simulink model "SysErrorDetect"  (R2019a)
settings: Solver=VariableStepAuto  StartTime=0.0  StopTime=10.0  RelTol=1e-3
settings Model: Creator=arsp2701  LastModifiedBy=arsp2701

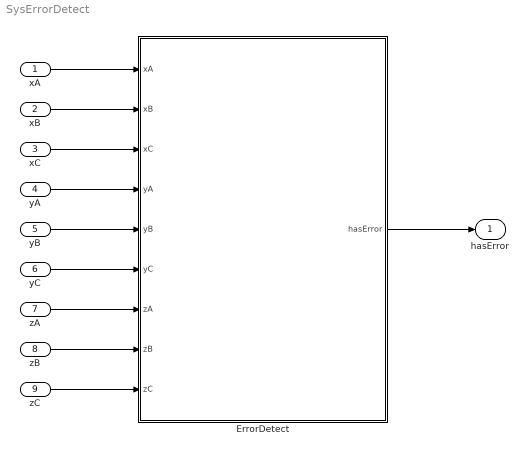
== system SysErrorDetect ==
  xA : Inport
  xB : Inport  Port=2
  xC : Inport  Port=3
  yA : Inport  Port=4
  yB : Inport  Port=5
  yC : Inport  Port=6
  zA : Inport  Port=7
  zB : Inport  Port=8
  zC : Inport  Port=9
  ErrorDetect : MATLAB Function  TreatAsAtomicUnit=on
  hasError : Outport
  wires:
  ErrorDetect/1(hasError) -> hasError/1
  xA/1 -> ErrorDetect/1(xA)
  xB/1 -> ErrorDetect/2(xB)
  xC/1 -> ErrorDetect/3(xC)
  yA/1 -> ErrorDetect/4(yA)
  yB/1 -> ErrorDetect/5(yB)
  yC/1 -> ErrorDetect/6(yC)
  zA/1 -> ErrorDetect/7(zA)
  zB/1 -> ErrorDetect/8(zB)
  zC/1 -> ErrorDetect/9(zC)

== matlab function SysErrorDetect/ErrorDetect ==
  data: xA input; xB input; hasError output; xC input; yA input; yB input; yC input; zA input; zB input; zC input
function hasError = ErrorDetect(xA, xB, xC, yA, yB, yC, zA, zB, zC)
    % Compute phi and theta (page 23)
    T_ABC = [
        yA -xA 1;
        yB -xB 1;
        yC -xC 1;
    ];
    
    m = T_ABC \ [zA zB zC]';
    phi = m(1);
    theta = m(2);
    z = m(3);

    % Margins
    margeAngle = 5;
    minZ = 0;
    maxZ = 3e-3; % 0.003 meters
    
    errorCount = 0;
    
    if (theta <= -margeAngle || theta >= margeAngle)
        error('WARNING: theta is out of bound (theta +- %i°).', margeAngle);
        errorCount = errorCount + 1;
    end
    
    if (phi <= -margeAngle || phi >= margeAngle)
        error('WARNING: phi is out of bound (phi +- %i°).', margeAngle);
        errorCount = errorCount + 1;
    end
    
    if (zA <= minZ || zA >= maxZ)
        error('WARNING: zA is out of bound (%.3f <= zA <= %.3f).', minZ, maxZ);
        errorCount = errorCount + 1;
    end
    
    if (zB <= minZ || zB >= maxZ)
        error('WARNING: zB is out of bound (%.3f <= zB <= %.3f).', minZ, maxZ);
        errorCount = errorCount + 1;
    end
    
    if (zC <= minZ || zC >= maxZ)
        error('WARNING: zC is out of bound (%.3f <= zC <= %.3f).', minZ, maxZ);
        errorCount = errorCount + 1;
    end
    
    hasError = errorCount > 0;
end
